simulink model "POWER_SYSTEM_FULL"  (R2025a)
settings: Solver=ode23t  StartTime=0  StopTime=5  FixedStep=1e-06  MinStep=1e-06  AbsTol=1e-6
model workspace (MAT data in the model file):
  CONTROL_INI.VSMP.PARAM.H = [15.5890205501 15.5890205501 15.5890205501 15.5890205501]
  CONTROL_INI.VSMP.PARAM.Dp = [20 20 20 20]
  CONTROL_INI.VSMP.PARAM.Dd = [0.156477821214 0.156477821214 0.156477821214 0.156477821214]
  CONTROL_INI.VSMP.PARAM.der2error = [1 1 1 1]
  CONTROL_INI.VSMP.TARGET.P_ref = [0.728496137496 0.728496137496 0.734176903563 0.734176903563]
  CONTROL_INI.VSMP.INPUT.P = [0.728496137496 0.728496137496 0.734176903563 0.734176903563]
  CONTROL_INI.VSMP.OUTPUT.w_pu = [1 1 1 1]
  CONTROL_INI.VSMP.OUTPUT.dth = [1 1 1 1]
  CONTROL_INI.VSMP.OUTPUT.th = [-0.655727257168 -0.655727257168 -0.596773515436 -0.596773515436]
  CONTROL_INI.VSMP.OUTPUT.MV = [20 20 20 20]
  CONTROL_INI.VSMP.STATE = [1  1  1  1; -0.655727257168  -0.655727257168  -0.596773515436  -0.596773515436]
  CONTROL_INI.VSMQ.PARAM.K_Fs_ref = [0.00177246709622 0.00177246709622 0.00177246709622 0.00177246709622]
  CONTROL_INI.VSMQ.PARAM.K_droopQV = [0.295235933108 0.295235933108 0.295235933108 0.295235933108]
  CONTROL_INI.VSMQ.TARGET.Vs_ref = [1 1 1 1]
  CONTROL_INI.VSMQ.TARGET.Q_ref = [0.279528149911 0.279528149911 0.34680626227 0.34680626227]
  CONTROL_INI.VSMQ.INPUT.Vs = [1.03097478396 1.03097478396 1.06643947684 1.06643947684]
  CONTROL_INI.VSMQ.INPUT.Q = [0.270383280666 0.270383280666 0.32719094133 0.32719094133]
  CONTROL_INI.VSMQ.OUTPUT.Fs_ref = [1.070537678 1.070537678 1.11055988863 1.11055988863]
  CONTROL_INI.VSMQ.OUTPUT.MV = [0 0 0 0]
  CONTROL_INI.VSMQ.STATE = [1.070537678 1.070537678 1.11055988863 1.11055988863]
  CONTROL_INI.RSCd.PARAM.Kp = [26.2007936931 26.2007936931 26.2007936931 26.2007936931]
  CONTROL_INI.RSCd.PARAM.Ki = [11667.9331248 11667.9331248 11667.9331248 11667.9331248]
  CONTROL_INI.RSCd.PARAM.b = [1 1 1 1]
  CONTROL_INI.RSCd.TARGET.iRSCd_ref = [1.07624735715 1.07624735715 1.16545801889 1.16545801889]
  CONTROL_INI.RSCd.INPUT.iRSCd = [1.07624735715 1.07624735715 1.16545801889 1.16545801889]
  CONTROL_INI.RSCd.OUTPUT.vRSCd = [0.0171862723129 0.0171862723129 0.0176580541869 0.0176580541869]
  CONTROL_INI.RSCd.OUTPUT.MV = [-0.00184970943607 -0.00184970943607 -0.00100750664806 -0.00100750664806]
  CONTROL_INI.RSCd.STATE = [-0.00184970943607 -0.00184970943607 -0.00100750664806 -0.00100750664806]
  CONTROL_INI.RSCq.PARAM.Kp = [26.9584626879 26.9584626879 26.9584626879 26.9584626879]
  CONTROL_INI.RSCq.PARAM.Ki = [11726.8571581 11726.8571581 11726.8571581 11726.8571581]
  CONTROL_INI.RSCq.PARAM.b = [1 1 1 1]
  CONTROL_INI.RSCq.TARGET.iRSCq_ref = [1.05756781089 1.05756781089 1.02646278241 1.02646278241]
  CONTROL_INI.RSCq.INPUT.iRSCq = [1.05756781089 1.05756781089 1.02646278241 1.02646278241]
  CONTROL_INI.RSCq.OUTPUT.vRSCq = [-0.142921611261 -0.142921611261 -0.1508739187 -0.1508739187]
  CONTROL_INI.RSCq.OUTPUT.MV = [-0.123549401898 -0.123549401898 -0.129680819521 -0.129680819521]
  CONTROL_INI.RSCq.STATE = [-0.123549401898 -0.123549401898 -0.129680819521 -0.129680819521]
  CONTROL_INI.VDC.PARAM.Kp = [0.0696845800453 0.0696845800453 0.0696845800453 0.0696845800453]
  CONTROL_INI.VDC.PARAM.Ki = [3.07602140958 3.07602140958 3.07602140958 3.07602140958]
  CONTROL_INI.VDC.PARAM.b = [1 1 1 1]
  CONTROL_INI.VDC.TARGET.Vdc2_ref = [1 1 1 1]
  CONTROL_INI.VDC.INPUT.Vdc2 = [1 1 1 1]
  CONTROL_INI.VDC.OUTPUT.Pg_ref = [-0.0767620514712 -0.0767620514712 -0.0776825582306 -0.0776825582306]
  CONTROL_INI.VDC.OUTPUT.MV = [-0.0767620514712 -0.0767620514712 -0.0776825582306 -0.0776825582306]
  CONTROL_INI.VDC.STATE = [-0.0767620514712 -0.0767620514712 -0.0776825582306 -0.0776825582306]
  CONTROL_INI.GSCd.PARAM.Kp = [0.322083043505 0.322083043505 0.322083043505 0.322083043505]
  CONTROL_INI.GSCd.PARAM.Ki = [127.577686075 127.577686075 127.577686075 127.577686075]
  CONTROL_INI.GSCd.PARAM.b = [1 1 1 1]
  CONTROL_INI.GSCd.TARGET.Qg_ref = [0 0 0 0]
  CONTROL_INI.GSCd.TARGET.iGSCd_ref = [0 0 0 0]
  CONTROL_INI.GSCd.INPUT.iGSCd = [-3.10168557505e-15 -3.10168557505e-15 -6.80011602583e-16 -6.80011602583e-16]
  CONTROL_INI.GSCd.OUTPUT.vGSCd = [0.0708413035779 0.0708413035779 0.0682389112282 0.0682389112282]
  CONTROL_INI.GSCd.OUTPUT.MV = [2.34814861689e-15 2.34814861689e-15 -1.1167396054e-15 -1.1167396054e-15]
  CONTROL_INI.GSCd.STATE = [2.34814861689e-15 2.34814861689e-15 -1.1167396054e-15 -1.1167396054e-15]
  CONTROL_INI.GSCq.PARAM.Kp = [0.336796601445 0.336796601445 0.336796601445 0.336796601445]
  CONTROL_INI.GSCq.PARAM.Ki = [112.607832611 112.607832611 112.607832611 112.607832611]
  CONTROL_INI.GSCq.PARAM.b = [1 1 1 1]
  CONTROL_INI.GSCq.TARGET.iGSCq_ref = [-0.128961227093 -0.128961227093 -0.126167626611 -0.126167626611]
  CONTROL_INI.GSCq.INPUT.iGSCq = [-0.128961227093 -0.128961227093 -0.126167626611 -0.126167626611]
  CONTROL_INI.GSCq.OUTPUT.vGSCq = [1.02862401667 1.02862401667 1.06435180834 1.06435180834]
  CONTROL_INI.GSCq.OUTPUT.MV = [-0.000289354764585 -0.000289354764585 -0.000283086666596 -0.000283086666596]
  CONTROL_INI.GSCq.STATE = [-0.000289354764585 -0.000289354764585 -0.000283086666596 -0.000283086666596]
  CONTROL_INI.VIMP.PARAM.Lv_pu = [0.06507 0.06507 0.06507 0.06507]
  CONTROL_INI.VIMP.PARAM.Rv_pu = [0 0 0 0]
  MODEL_INI.PARAM.SIM_SAMPLING_TIME = 1e-06
  MODEL_INI.PARAM.SIM_FINAL_TIME = 5
  MODEL_INI.BASE.Ub = 690
  MODEL_INI.BASE.Ib = 1760
  MODEL_INI.BASE.Sb = 2103402.50071
  MODEL_INI.BASE.Zb = 0.392045454545
  MODEL_INI.BASE.f0 = 50
  MODEL_INI.BASE.fbase = 50
  MODEL_INI.BASE.wbase = 314.159265359
  MODEL_INI.BASE.Lb = 0.00124791944015
  MODEL_INI.BASE.Cb = 0.00811920869106
  MODEL_INI.DFIG.PARAM.nDFIG = 4
  MODEL_INI.DFIG.PARAM.p = [2 2 2 2]
  MODEL_INI.DFIG.PARAM.WMECm = [157.079632679 157.079632679 157.079632679 157.079632679]
  MODEL_INI.DFIG.PARAM.WMECe = [314.159265359 314.159265359 314.159265359 314.159265359]
  MODEL_INI.DFIG.PARAM.Lsig_s_H = [8.7e-05 8.7e-05 8.7e-05 8.7e-05]
  MODEL_INI.DFIG.PARAM.Lsig_r_H = [8.7e-05 8.7e-05 8.7e-05 8.7e-05]
  MODEL_INI.DFIG.PARAM.Lm_H = [0.0025 0.0025 0.0025 0.0025]
  MODEL_INI.DFIG.PARAM.Ls_H = [0.002587 0.002587 0.002587 0.002587]
  MODEL_INI.DFIG.PARAM.Lr_H = [0.002587 0.002587 0.002587 0.002587]
  MODEL_INI.DFIG.PARAM.sigma = [0.0661284179513 0.0661284179513 0.0661284179513 0.0661284179513]
  MODEL_INI.DFIG.PARAM.Rs_Ohm = [0.0026 0.0026 0.0026 0.0026]
  MODEL_INI.DFIG.PARAM.Rr_Ohm = [0.0029 0.0029 0.0029 0.0029]
  MODEL_INI.DFIG.PARAM.Rc_Ohm = [1000000 1000000 1000000 1000000]
  MODEL_INI.DFIG.PARAM.Ur_open_rotor_V = [2070 2070 2070 2070]
  MODEL_INI.DFIG.PARAM.Cdc = [0.00225 0.00225 0.00225 0.00225]
  MODEL_INI.DFIG.PARAM.SCR_transformer = [10 10 5 5]
  MODEL_INI.DFIG.PARAM.XR_transformer = [10 10 10 10]
  MODEL_INI.DFIG.PARAM.Lt_H = [7.20486624699e-05 7.20486624699e-05 0.00014409732494 0.00014409732494]
  MODEL_INI.DFIG.PARAM.Rt_Ohm = [0.00226347548716 0.00226347548716 0.00452695097433 0.00452695097433]
  MODEL_INI.DFIG.PARAM.Lfgsc_H = [2.8e-05 2.8e-05 2.8e-05 2.8e-05]
  MODEL_INI.DFIG.PARAM.Rfgsc_Ohm = [0.000879645943005 0.000879645943005 0.000879645943005 0.000879645943005]
  MODEL_INI.DFIG.PARAM.Lsig_s_pu = [0.0697160387127 0.0697160387127 0.0697160387127 0.0697160387127]
  MODEL_INI.DFIG.PARAM.Lsig_r_pu = [0.0697160387127 0.0697160387127 0.0697160387127 0.0697160387127]
  MODEL_INI.DFIG.PARAM.Lm_pu = [2.00333444577 2.00333444577 2.00333444577 2.00333444577]
  MODEL_INI.DFIG.PARAM.Ls_pu = [2.07305048448 2.07305048448 2.07305048448 2.07305048448]
  MODEL_INI.DFIG.PARAM.Lr_pu = [2.07305048448 2.07305048448 2.07305048448 2.07305048448]
  MODEL_INI.DFIG.PARAM.sigma_pu = [0.0661284179513 0.0661284179513 0.0661284179513 0.0661284179513]
  MODEL_INI.DFIG.PARAM.Rs_pu = [0.00663188405797 0.00663188405797 0.00663188405797 0.00663188405797]
  MODEL_INI.DFIG.PARAM.Rr_pu = [0.00739710144928 0.00739710144928 0.00739710144928 0.00739710144928]
  MODEL_INI.DFIG.PARAM.Rc_pu = [2550724.63768 2550724.63768 2550724.63768 2550724.63768]
  MODEL_INI.DFIG.PARAM.Rfe_pu = [2550724.63768 2550724.63768 2550724.63768 2550724.63768]
  MODEL_INI.DFIG.PARAM.Ur_open_rotor_pu = [3 3 3 3]
  MODEL_INI.DFIG.PARAM.Cdc_pu = 0.483918802711
  MODEL_INI.DFIG.PARAM.Lt_pu = [0.057735026919 0.057735026919 0.115470053838 0.115470053838]
  MODEL_INI.DFIG.PARAM.Rt_pu = [0.0057735026919 0.0057735026919 0.0115470053838 0.0115470053838]
  MODEL_INI.DFIG.PARAM.Lfgsc_pu = [0.0224373457926 0.0224373457926 0.0224373457926 0.0224373457926]
  MODEL_INI.DFIG.PARAM.Rfgsc_pu = [0.00224373457926 0.00224373457926 0.00224373457926 0.00224373457926]
  MODEL_INI.DFIG.PARAM.J = [2.53 2.53 2.53 2.53]
  MODEL_INI.DFIG.PARAM.Jt_kgm2 = [800 800 800 800]
  MODEL_INI.DFIG.PARAM.Dt_Nms_rad = [0.1 0.1 0.1 0.1]
  MODEL_INI.DFIG.PARAM.Ktg_Nm_rad = [12500 12500 12500 12500]
  MODEL_INI.DFIG.PARAM.Dtg_Nms_rad = [130 130 130 130]
  MODEL_INI.DFIG.PARAM.Jg_kgm2 = [90 90 90 90]
  MODEL_INI.DFIG.PARAM.Dg_Nms_rad = [0.1 0.1 0.1 0.1]
  MODEL_INI.DFIG.PARAM.Ht_pu = [4.69220912201 4.69220912201 4.69220912201 4.69220912201]
  MODEL_INI.DFIG.PARAM.Dt_pu = [0.0011730522805 0.0011730522805 0.0011730522805 0.0011730522805]
  MODEL_INI.DFIG.PARAM.Hg_pu = [0.527873526226 0.527873526226 0.527873526226 0.527873526226]
  MODEL_INI.DFIG.PARAM.Dg_pu = [0.0011730522805 0.0011730522805 0.0011730522805 0.0011730522805]
  MODEL_INI.DFIG.PARAM.Dtg_pu = [1.52496796465 1.52496796465 1.52496796465 1.52496796465]
  MODEL_INI.DFIG.PARAM.Ktg_pu = [0.933485344735 0.933485344735 0.933485344735 0.933485344735]
  MODEL_INI.DFIG.PARAM.turbineData.ratedTurbinePower = 2000000
  MODEL_INI.DFIG.PARAM.turbineData.ratedTurbineSpeed = 2.80648943721
  MODEL_INI.DFIG.PARAM.turbineData.ratedWindSpeed = 12.5
  MODEL_INI.DFIG.PARAM.turbineData.turbineRadius = 35
  MODEL_INI.DFIG.PARAM.turbineData.airDensity = 1.225
  MODEL_INI.DFIG.PARAM.turbineData.Cp_coeff_matrix = [-0.533799944678  0.284966457097  -0.0246612463409  0.00070387634662  -6.19435778221e-06; 0.0502347840223  -0.0141180188397  0.000236959314197  9.72360914257e-05  -3.95863369447e-06; -0.0141053149856  0.00789606939988  -0.0013835145015  8.1445517726e-05  -1.33347929886e-06; 0.00189515235857  -0.00115030050123  0.000206019398382  -1.24987823414e-05  1.58554758305e-07; -7.04963027946e-05  4.2809340349e-05  -7.43463233727e-06  4.06348518101e-07  -2.85640254235e-09]
  MODEL_INI.DFIG.BASE.Udc_base = [1200 1200 1200 1200]
  MODEL_INI.DFIG.BASE.Idc_base = [1752.83541726 1752.83541726 1752.83541726 1752.83541726]
  MODEL_INI.DFIG.BASE.Zdc_base = [0.68460506228 0.68460506228 0.68460506228 0.68460506228]
  MODEL_INI.DFIG.BASE.Cdc_base = [0.00464954035139 0.00464954035139 0.00464954035139 0.00464954035139]
  MODEL_INI.DFIG.BASE.wmbase = [157.079632679 157.079632679 157.079632679 157.079632679]
  MODEL_INI.DFIG.BASE.Tebase = [13390.676212 13390.676212 13390.676212 13390.676212]
  MODEL_INI.DFIG.BASE.Jb = [85.2476924193 85.2476924193 85.2476924193 85.2476924193]
  MODEL_INI.DFIG.INPUT.vPCC_r = [0.714142842854 0.714142842854 0.714142842854 0.714142842854]
  MODEL_INI.DFIG.INPUT.vPCC_i = [0.7 0.7 0.7 0.7]
  MODEL_INI.DFIG.INPUT.vRSC_r = [-0.0735225072874 -0.0735225072874 -0.0701816981017 -0.0701816981017]
  MODEL_INI.DFIG.INPUT.vRSC_i = [-0.123759427292 -0.123759427292 -0.134719246855 -0.134719246855]
  MODEL_INI.DFIG.INPUT.vGSC_r = [0.683338070975 0.683338070975 0.654584845977 0.654584845977]
  MODEL_INI.DFIG.INPUT.vGSC_i = [0.772097752046 0.772097752046 0.842033253697 0.842033253697]
  MODEL_INI.DFIG.INPUT.windSpeed = [11.0080618911 11.0080618911 11.0368315613 11.0368315613]
  MODEL_INI.DFIG.INPUT.turbinePitch = [1 1 1 1]
  MODEL_INI.DFIG.OUTPUT.vs_r = [0.68545508048 0.68545508048 0.656767318105 0.656767318105]
  MODEL_INI.DFIG.OUTPUT.vs_i = [0.770104108417 0.770104108417 0.840208216834 0.840208216834]
  MODEL_INI.DFIG.OUTPUT.is_r = [-1.07438763375 -1.07438763375 -1.0821166602 -1.0821166602]
  MODEL_INI.DFIG.OUTPUT.is_i = [-0.50997333627 -0.50997333627 -0.507828664614 -0.507828664614]
  MODEL_INI.DFIG.OUTPUT.ir_r = [1.4978757059 1.4978757059 1.5408603146 1.5408603146]
  MODEL_INI.DFIG.OUTPUT.ir_i = [0.182006642923 0.182006642923 0.194081756892 0.194081756892]
  MODEL_INI.DFIG.OUTPUT.ig_r = [-0.0786322810944 -0.0786322810944 -0.0709032546372 -0.0709032546372]
  MODEL_INI.DFIG.OUTPUT.ig_i = [-0.102215275098 -0.102215275098 -0.104359946754 -0.104359946754]
  MODEL_INI.DFIG.OUTPUT.it_r = [1.15301991484 1.15301991484 1.15301991484 1.15301991484]
  MODEL_INI.DFIG.OUTPUT.it_i = [0.612188611368 0.612188611368 0.612188611368 0.612188611368]
  MODEL_INI.DFIG.OUTPUT.Vdc = [1 1 1 1]
  MODEL_INI.DFIG.OUTPUT.P_GSC = [-0.076587023214 -0.076587023214 -0.0775304863749 -0.0775304863749]
  MODEL_INI.DFIG.OUTPUT.P_RSC = [-0.0765870232066 -0.0765870232066 -0.0775304863727 -0.0775304863727]
  MODEL_INI.DFIG.OUTPUT.Pdc = [-7.36979921534e-12 -7.36979921534e-12 -2.18218498826e-12 -2.18218498826e-12]
  MODEL_INI.DFIG.OUTPUT.wr = [1.13130130564 1.13130130564 1.13264773079 1.13264773079]
  MODEL_INI.DFIG.OUTPUT.Pm = [0.746659273078 0.746659273078 0.752978959715 0.752978959715]
  MODEL_INI.DFIG.STATE = [0.706916556634  0.706916556634  0.710436806016  0.710436806016; -0.727925020657  -0.727925020657  -0.734633242246  -0.734633242246; 0.952814203022  0.952814203022  1.02643964198  1.02643964198; -0.644338191682  -0.644338191682  -0.615009376214  -0.615009376214; 1.13130130564  1.13130130564  1.13264773079  1.13264773079; 1  1  1  1; -0.0683339355027  -0.0683339355027  -0.134730152485  -0.134730152485; -0.0376381654294  -0.0376381654294  -0.0730310121258  -0.0730310121258; 1.13130130564  1.13130130564  1.13264773079  1.13264773079; 0.658673288027  0.658673288027  0.663466708323  0.663466708323]
  MODEL_INI.LINE.PARAM.nLINE = 1
  MODEL_INI.LINE.PARAM.R_pu = 1e-05
  MODEL_INI.LINE.PARAM.L_pu = 1e-05
  MODEL_INI.LINE.PARAM.Rn1_pu = 100
  MODEL_INI.LINE.PARAM.Cn1_pu = 0.001
  MODEL_INI.LINE.PARAM.Rn2_pu = 100
  MODEL_INI.LINE.PARAM.Cn2_pu = 0.001
  MODEL_INI.LINE.PARAM.load_node = 2
  MODEL_INI.LINE.INPUT.in1_r = 4.61207965936
  MODEL_INI.LINE.INPUT.in1_i = 2.44875444547
  MODEL_INI.LINE.INPUT.in2_r = 4.60563823093
  MODEL_INI.LINE.INPUT.in2_i = 2.44104030263
  MODEL_INI.LINE.INPUT.il1_r = 0
  MODEL_INI.LINE.INPUT.il1_i = 0
  MODEL_INI.LINE.INPUT.il2_r = 0
  MODEL_INI.LINE.INPUT.il2_i = 0
  MODEL_INI.LINE.OUTPUT.vn1_r = 0.714142842854
  MODEL_INI.LINE.OUTPUT.vn1_i = 0.7
  MODEL_INI.LINE.OUTPUT.Vpcc = 1
  MODEL_INI.LINE.OUTPUT.vn2_r = 1
  MODEL_INI.LINE.OUTPUT.vn2_i = 0
  MODEL_INI.LINE.OUTPUT.i_r = 4.60563823093
  MODEL_INI.LINE.OUTPUT.i_i = 2.44104030263
  MODEL_INI.LINE.STATE = [4.60563823093; 2.44104030263; 0.714142842854; 0.7; 1; 0]
  MODEL_INI.GRID.PARAM.nGRID = 1
  MODEL_INI.GRID.PARAM.SCR_grid = 1
  MODEL_INI.GRID.PARAM.XR_grid = 10
  MODEL_INI.GRID.PARAM.Lg_H = 0.000180121656175
  MODEL_INI.GRID.PARAM.Rg_Ohm = 0.00565868871791
  MODEL_INI.GRID.PARAM.Lg_pu = 0.144337567297
  MODEL_INI.GRID.PARAM.Rg_pu = 0.0144337567297
  MODEL_INI.GRID.PARAM.Deq_pu = 20
  MODEL_INI.GRID.PARAM.Tgov = 0.2
  MODEL_INI.GRID.PARAM.Ttb1 = 0.3
  MODEL_INI.GRID.PARAM.Ttb2 = 7
  MODEL_INI.GRID.PARAM.H = 5
  MODEL_INI.GRID.BASE.Ub = 690
  MODEL_INI.GRID.BASE.Sb = 8413610.00285
  MODEL_INI.GRID.INPUT.v_grid_r = 1
  MODEL_INI.GRID.INPUT.v_grid_i = 0
  MODEL_INI.GRID.INPUT.Pg_ref = -0.664766618104
  MODEL_INI.GRID.OUTPUT.f_pu = 1
  MODEL_INI.GRID.OUTPUT.Pmech = -0.664766618104
  MODEL_INI.GRID.OUTPUT.Pgrid = -0.664766618104
  MODEL_INI.GRID.OUTPUT.Qgrid = 0.352333818956
  MODEL_INI.GRID.STATE = [-0.664766618104; -0.664766618104; 0; 1]
  initialMemoryState = [1.15301991484; 1.15301991484; 1.15301991484; 1.15301991484; 0.612188611368; 0.612188611368; 0.612188611368; 0.612188611368; -1.07438763375; -1.07438763375; -1.0821166602; -1.0821166602; -0.50997333627; -0.50997333627; -0.507828664614; -0.507828664614; 1.4978757059; 1.4978757059; 1.5408603146; 1.5408603146; 0.182006642923; 0.182006642923; 0.194081756892; 0.194081756892; 0.68545508048; 0.68545508048; 0.656767318105; 0.656767318105; 0.770104108417; 0.770104108417; 0.840208216834; 0.840208216834; 1; 1; 1; 1; 1.13130130564; 1.13130130564; 1.13264773079; 1.13264773079]
undefined symbols (not defined in the file or in its folder): CONTROL, MODEL, monitorDFIG, pref_mask_vec, qref_mask_vec
(part 1 of 3)
settings SolverCC: SolverResetMethod=Robust
settings DataIOCC: LimitDataPoints=on  MaxDataPoints=1  SaveFinalState=on  SaveFormat=StructureWithTime  SaveOutput=off  SignalLogging=off  DSMLogging=off  SaveTime=off  ReturnWorkspaceOutputs=off
settings OptimizationCC: BlockReduction=off  OptimizeBlockIOStorage=off  BufferReuse=off
settings DebuggingCC: AlgebraicLoopMsg=none  ArtificialAlgebraicLoopMsg=none
settings ModelReferenceCC: EnableRefExpFcnMdlSchedulingChecks=on
settings RTWCC: GPUComputeCapability=3.5

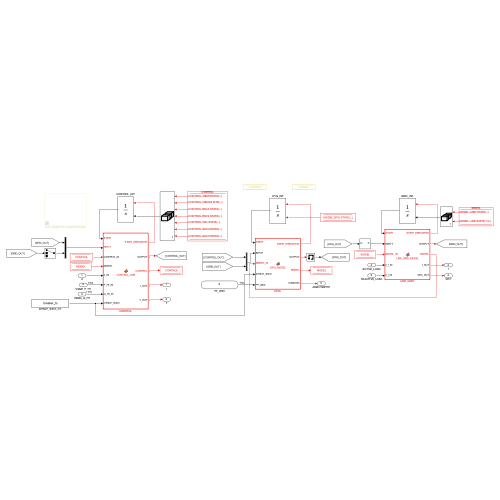
[thumbnail: Simulink's stored preview of the top-level diagram]
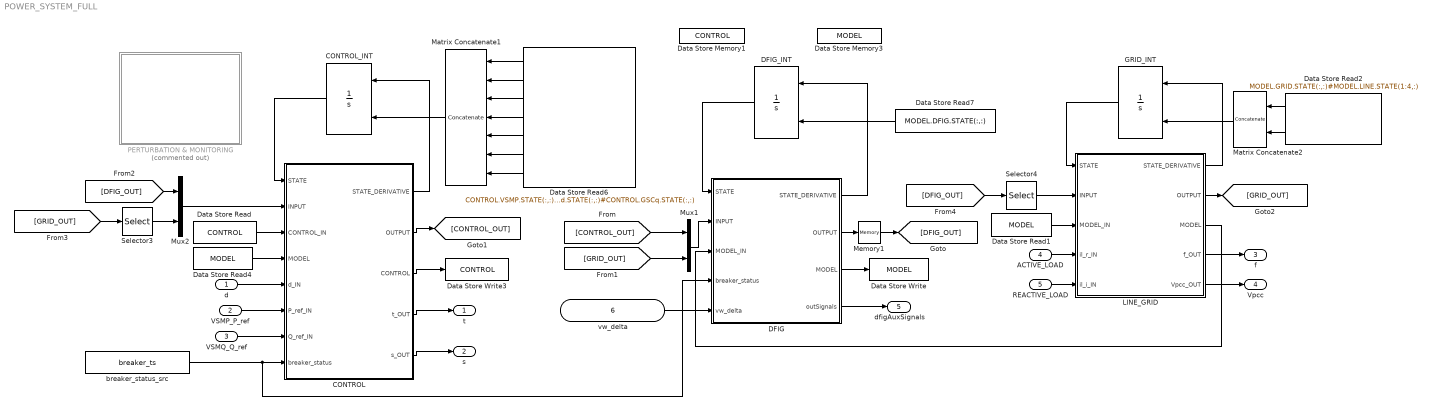
== system POWER_SYSTEM_FULL ==
  d : Inport
  VSMP_P_ref : Inport  Port=2  PortDimensions=[1 MODEL_INI.DFIG.PARAM.nDFIG]
  VSMQ_Q_ref : Inport  Port=3  PortDimensions=[1 MODEL_INI.DFIG.PARAM.nDFIG]
  ACTIVE_LOAD : Inport  Port=4  PortDimensions=1
  REACTIVE_LOAD : Inport  Port=5  PortDimensions=1
  vw_delta : Inport  Port=6  PortDimensions=[1 4]
  CONTROL : MATLAB Function  TreatAsAtomicUnit=on
  CONTROL_INT : Integrator  InitialConditionSource=external
  DFIG : MATLAB Function  TreatAsAtomicUnit=on
  DFIG_INT : Integrator  InitialConditionSource=external
  Data Store Memory1 : DataStoreMemory  Priority=2  DataStoreName=CONTROL  ReadBeforeWriteMsg=warning  WriteAfterWriteMsg=warning  WriteAfterReadMsg=warning  InitialValue=CONTROL_INI  ShowAdditionalParam=off  OutDataTypeStr=Bus: CONTROL_Bus
  Data Store Memory3 : DataStoreMemory  Priority=2  DataStoreName=MODEL  ReadBeforeWriteMsg=warning  WriteAfterWriteMsg=warning  WriteAfterReadMsg=warning  InitialValue=MODEL_INI  ShowAdditionalParam=off  OutDataTypeStr=Bus: MODEL_Bus
  Data Store Read : DataStoreRead  DataStoreName=CONTROL  IndexOptions=Index vector (dialog)  Indices=1  OutputSizes=1
  Data Store Read1 : DataStoreRead  DataStoreName=MODEL  IndexOptions=Index vector (dialog)  Indices=1  OutputSizes=1
  Data Store Read2 : DataStoreRead  DataStoreName=MODEL  DataStoreElements=MODEL.GRID.STATE(:,:)#MODEL.LINE.STATE(1:4,:)  IndexOptions=Index vector (dialog)  Indices=1  OutputSizes=1
  Data Store Read4 : DataStoreRead  DataStoreName=MODEL  IndexOptions=Index vector (dialog)  Indices=1  OutputSizes=1
  Data Store Read6 : DataStoreRead  DataStoreName=CONTROL  DataStoreElements=CONTROL.VSMP.STATE(:,:)#CONTROL.VSMQ.STATE(:,:)#CONTROL.RSCd.STATE(:,:)#CONTROL.RSCq.STATE(:,:)#CONTROL.VDC.STATE(:,:)#CONTROL.GSCd.STATE(:,:)#CONTROL.GSCq.STATE(:,:)  IndexOptions=Index vector (dialog)  Indices=1  OutputSizes=1
  Data Store Read7 : DataStoreRead  DataStoreName=MODEL  DataStoreElements=MODEL.DFIG.STATE(:,:)  IndexOptions=Index vector (dialog)  Indices=1  OutputSizes=1
  Data Store Write : DataStoreWrite  DataStoreName=MODEL  IndexOptions=Index vector (dialog)  Indices=1  OutputSizes=1
  Data Store Write3 : DataStoreWrite  DataStoreName=CONTROL  IndexOptions=Index vector (dialog)  Indices=1  OutputSizes=1
  GRID_INT : Integrator  InitialConditionSource=external
  LINE_GRID : MATLAB Function  TreatAsAtomicUnit=on
  Matrix Concatenate1 : Concatenate  NumInputs=7  Mode=Multidimensional array
  Matrix Concatenate2 : Concatenate  Mode=Multidimensional array
  Memory1 : Memory  InitialCondition=initialMemoryState  LinearizeMemory=on
  Mux1 : Mux  Inputs=2
  Mux2 : Mux  Inputs=2
  PERTURBATION & MONITORING : Subsystem  Priority=40  Commented=on
  Selector3 : Selector  InputPortWidth=3  IndexOptions=Index vector (dialog)  Indices=1  OutputSizes=1
  Selector4 : Selector  InputPortWidth=10*MODEL_INI.DFIG.PARAM.nDFIG  IndexOptions=Index vector (dialog)  Indices=1:8  OutputSizes=1
  breaker_status_src : FromWorkspace  VariableName=breaker_ts  Interpolate=off  OutputAfterFinalValue=Holding final value
  t : Outport
  s : Outport  Port=2
  f : Outport  Port=3
  Vpcc : Outport  Port=4
  dfigAuxSignals : Outport  Port=5
  wires:
  Data Store Read7/1 -> DFIG_INT/2
  DFIG_INT/1 -> DFIG/1(STATE)
  DFIG/1(STATE_DERIVATIVE) -> DFIG_INT/1
  DFIG/3(MODEL) -> Data Store Write/1
  GRID_INT/1 -> LINE_GRID/1(STATE)
  LINE_GRID/1(STATE_DERIVATIVE) -> GRID_INT/1
  CONTROL_INT/1 -> CONTROL/1(STATE)
  CONTROL/3(CONTROL) -> Data Store Write3/1
  Matrix Concatenate1/1 -> CONTROL_INT/2
  Data Store Read/1 -> CONTROL/3(CONTROL_IN)
  d/1 -> CONTROL/5(d_IN)
  CONTROL/4(t_OUT) -> t/1
  CONTROL/5(s_OUT) -> s/1
  Data Store Read6/1 -> Matrix Concatenate1/1
  Data Store Read6/2 -> Matrix Concatenate1/2
  Data Store Read6/3 -> Matrix Concatenate1/3
  Data Store Read6/4 -> Matrix Concatenate1/4
  Data Store Read6/5 -> Matrix Concatenate1/5
  Data Store Read6/6 -> Matrix Concatenate1/6
  Data Store Read6/7 -> Matrix Concatenate1/7
  VSMQ_Q_ref/1 -> CONTROL/7(Q_ref_IN)
  ACTIVE_LOAD/1 -> LINE_GRID/4(il_r_IN)
  REACTIVE_LOAD/1 -> LINE_GRID/5(il_i_IN)
  LINE_GRID/4(f_OUT) -> f/1
  LINE_GRID/5(Vpcc_OUT) -> Vpcc/1
  LINE_GRID/3(MODEL) -> DFIG/3(MODEL_IN)
  DFIG/2(OUTPUT) -> Memory1/1
  CONTROL/2(OUTPUT) -> [CONTROL_OUT]
  [CONTROL_OUT] -> Mux1/1
  [GRID_OUT] -> Mux1/2
  [DFIG_OUT] -> Mux2/1
  [GRID_OUT] -> Selector3/1
  Selector3/1 -> Mux2/2
  [DFIG_OUT] -> Selector4/1
  Data Store Read4/1 -> CONTROL/4(MODEL)
  Selector4/1 -> LINE_GRID/2(INPUT)
  Mux1/1 -> DFIG/2(INPUT)
  Mux2/1 -> CONTROL/2(INPUT)
  CONTROL/1(STATE_DERIVATIVE) -> CONTROL_INT/1
  LINE_GRID/2(OUTPUT) -> [GRID_OUT]
  Memory1/1 -> [DFIG_OUT]
  VSMP_P_ref/1 -> CONTROL/6(P_ref_IN)
  Data Store Read1/1 -> LINE_GRID/3(MODEL_IN)
  Data Store Read2/1 -> Matrix Concatenate2/1
  Data Store Read2/2 -> Matrix Concatenate2/2
  Matrix Concatenate2/1 -> GRID_INT/2
  DFIG/4(outSignals) -> dfigAuxSignals/1
  breaker_status_src/1 -> DFIG/4(breaker_status), CONTROL/8(breaker_status)
  vw_delta/1 -> DFIG/5(vw_delta)

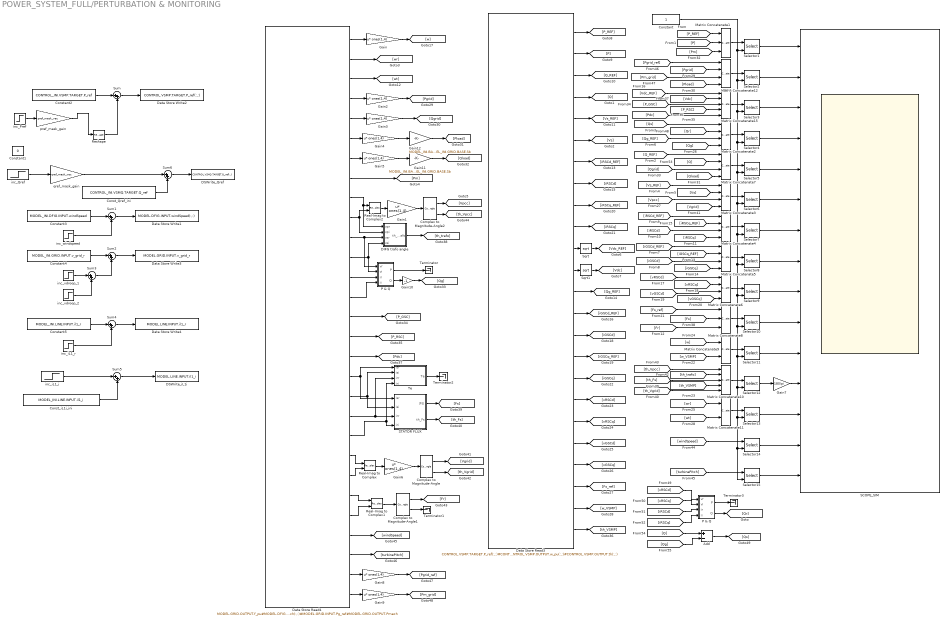
== system POWER_SYSTEM_FULL/PERTURBATION & MONITORING ==
  Add : Sum  Inputs=+-
  Complex to Magnitude-Angle : ComplexToMagnitudeAngle
  Complex to Magnitude-Angle1 : ComplexToMagnitudeAngle
  Complex to Magnitude-Angle2 : ComplexToMagnitudeAngle
  Const_Qref_ini : Constant  Value=CONTROL_INI.VSMQ.TARGET.Q_ref  SampleTime=-1
  Const_iL1i_ini : Constant  Value=MODEL_INI.LINE.INPUT.il1_i  SampleTime=-1
  Constant : Constant
  Constant1 : Constant  Value=0  VectorParams1D=off  SampleTime=-1
  Constant2 : Constant  Value=CONTROL_INI.VSMP.TARGET.P_ref  SampleTime=-1
  Constant3 : Constant  Value=MODEL_INI.DFIG.INPUT.windSpeed  SampleTime=-1
  Constant4 : Constant  Value=MODEL_INI.GRID.INPUT.v_grid_r  SampleTime=-1
  Constant5 : Constant  Value=MODEL_INI.LINE.INPUT.il1_r  SampleTime=-1
  DIFG trafo angle : Subsystem
  DSWrite_Qref : DataStoreWrite  DataStoreName=CONTROL  DataStoreElements=CONTROL.VSMQ.TARGET.Q_ref(:,:)  IndexOptions=Index vector (dialog)  Indices=1  OutputSizes=1
  DSWrite_iL1i : DataStoreWrite  DataStoreName=MODEL  DataStoreElements=MODEL.LINE.INPUT.il1_i  IndexOptions=Index vector (dialog)  Indices=1  OutputSizes=1
  Data Store Read3 : DataStoreRead  DataStoreName=CONTROL  DataStoreElements=CONTROL.VSMP.TARGET.P_ref(:,:)#CONTROL.VSMP.INPUT.P(:,:)#CONTROL.VSMQ.TARGET.Q_ref(:,:)#CONTROL.VSMQ.INPUT.Q(:,:)#CONTROL.VSMQ.TARGET.Vs_ref(:,:)#CONTROL.VSMQ.INPUT.Vs(:,:)#CONTROL.RSCd.TARGET.iRSCd_ref(:,:)#CONTROL.RSCd.INPUT.iRSCd(:,:)#CONTROL.RSCq.TARGET.iRSCq_ref(:,:)#CONTROL.RSCq.INPUT.iRSCq(:,:)#CONTROL.VDC.TARGET.Vdc2_ref(:,:)#CONTROL.VDC.INPUT.Vdc2(:,:)#CONTROL.GSCd.TARGET.Qg_ref(:,:)#CONTROL.GSCd.TARGET.iGSCd_ref(:,:)#CONTROL.GSCd.INPUT.iGSCd(:,:)#CONTROL.GSCq.TARGET.iGSCq_ref(:,:)#CONTROL.GSCq.INPUT.iGSCq(:,:)#CONTROL.RSCd.OUTPUT.vRSCd(:,:)#CONTROL.RSCq.OUTPUT.vRSCq(:,:)#CONTROL.GSCd.OUTPUT.vGSCd(:,:)#CONTROL.GSCq.OUTPUT.vGSCq(:,:)#CONTROL.VSMQ.OUTPUT.Fs_ref(:,:)#CONTROL.VSMP.OUTPUT.w_pu(:,:)#CONTROL.VSMP.OUTPUT.th(:,:)  IndexOptions=Index vector (dialog)  Indices=1  OutputSizes=1
  Data Store Read4 : DataStoreRead  DataStoreName=MODEL  DataStoreElements=MODEL.GRID.OUTPUT.f_pu#MODEL.DFIG.OUTPUT.wr(:,:)#MODEL.DFIG.STATE(9,:)#MODEL.GRID.OUTPUT.Pgrid#MODEL.GRID.OUTPUT.Qgrid#MODEL.LINE.INPUT.il1_r#MODEL.LINE.INPUT.il1_i#MODEL.DFIG.OUTPUT.Pm(:,:)#MODEL.LINE.OUTPUT.vn1_r#MODEL.LINE.OUTPUT.vn1_i#MODEL.DFIG.OUTPUT.vs_r(:,:)#MODEL.DFIG.OUTPUT.vs_i(:,:)#MODEL.DFIG.OUTPUT.ig_r(:,:)#MODEL.DFIG.OUTPUT.ig_i(:,:)#MODEL.DFIG.OUTPUT.P_GSC(:,:)#MODEL.DFIG.OUTPUT.P_RSC(:,:)#MODEL.DFIG.OUTPUT.Pdc(:,:)#MODEL.DFIG.OUTPUT.is_r(:,:)#MODEL.DFIG.OUTPUT.is_i(:,:)#MODEL.DFIG.OUTPUT.ir_r(:,:)#MODEL.DFIG.OUTPUT.ir_i(:,:)#MODEL.GRID.INPUT.v_grid_r#MODEL.GRID.INPUT.v_grid_i#MODEL.DFIG.STATE(3,:)#MODEL.DFIG.STATE(4,:)#MODEL.DFIG.INPUT.windSpeed(:,:)#MODEL.DFIG.INPUT.turbinePitch(:,:)#MODEL.GRID.INPUT.Pg_ref#MODEL.GRID.OUTPUT.Pmech  IndexOptions=Index vector (dialog)  Indices=1  OutputSizes=1
  Data Store Write1 : DataStoreWrite  DataStoreName=MODEL  DataStoreElements=MODEL.DFIG.INPUT.windSpeed(:,:)  IndexOptions=Index vector (dialog)  Indices=1  OutputSizes=1
  Data Store Write2 : DataStoreWrite  DataStoreName=CONTROL  DataStoreElements=CONTROL.VSMP.TARGET.P_ref(:,:)  IndexOptions=Index vector (dialog)  Indices=1  OutputSizes=1
  Data Store Write3 : DataStoreWrite  DataStoreName=MODEL  DataStoreElements=MODEL.GRID.INPUT.v_grid_r  IndexOptions=Index vector (dialog)  Indices=1  OutputSizes=1
  Data Store Write4 : DataStoreWrite  DataStoreName=MODEL  DataStoreElements=MODEL.LINE.INPUT.il1_r  IndexOptions=Index vector (dialog)  Indices=1  OutputSizes=1
  Gain{,1..6,8..9} (9 alike) : Gain  Gain=ones(1,4)  Multiplication=Matrix(u*K)
  Gain10 : Gain  Gain=-1
  Gain11 : Gain  Gain=MODEL_INI.BASE.Sb/MODEL_INI.GRID.BASE.Sb
  Gain12 : Gain  Gain=MODEL_INI.BASE.Sb/MODEL_INI.GRID.BASE.Sb
  Gain7 : Gain  Gain=180/pi
  Matrix Concatenate1 : Concatenate  NumInputs=3  Mode=Multidimensional array
  Matrix Concatenate10 : Concatenate  NumInputs=5  Mode=Multidimensional array
  Matrix Concatenate11 : Concatenate  Mode=Multidimensional array
  Matrix Concatenate{2..7,12} (7 alike) : Concatenate  NumInputs=4  Mode=Multidimensional array
  Matrix Concatenate15 : Concatenate  NumInputs=5  Mode=Multidimensional array
  Matrix Concatenate8 : Concatenate  NumInputs=3  Mode=Multidimensional array
  Matrix Concatenate9 : Concatenate  Mode=Multidimensional array
  P & Q : Subsystem
  "P & Q " : Subsystem
  Real-Imag to Complex : RealImagToComplex
  Real-Imag to Complex1 : RealImagToComplex
  Real-Imag to Complex2 : RealImagToComplex
  Reshape : Reshape  OutputDimensionality=Row vector (2-D)
  SCOPE_SIM : Scope  NumInputPorts=15
      settings: Title=DFIG ACTIVE POWER (pu)  ActiveDisplayYMinimum=0.70146460984873871  ActiveDisplayYMaximum=0.96691028131648715  DataLoggingVariableName=SCOPE_SIM
  STATOR FLUX : Subsystem
  Selector{1..15} (15 alike) : Selector  NumberOfDimensions=2  InputPortWidth=10  IndexOptions=Select all,Index vector (port)  Indices=monitorDFIG,1  OutputSizes=1,1
  Sqrt : Sqrt
  Sqrt1 : Sqrt
  Sum{,1..6} (7 alike) : Sum  Inputs=|++
  Te : Subsystem
  Terminator{,1..3} (4 alike) : Terminator
  inc_Pref : Step  After=0.2  SampleTime=0
  inc_Qref : Step  Time=999  After=0
  inc_iL1_i : Step  Time=999  After=0
  inc_iL1_r : Step  After=0.0  SampleTime=0
  inc_vdroop_1 : Step  After=0.0  SampleTime=0
  inc_vdroop_2 : Step  Time=1.5  After=0.0  SampleTime=0
  inc_windspeed : Step  After=0.0  SampleTime=0
  pref_mask_gain : Gain  Gain=pref_mask_vec
  qref_mask_gain : Gain  Gain=qref_mask_vec
  wires:
  Data Store Read3/2 -> [P]
  Data Store Read3/5 -> [Vs_REF]
  [P_REF] -> Matrix Concatenate1/1
  Data Store Read3/8 -> [iRSCd]
  Data Store Read3/4 -> [Q]
  Data Store Read3/7 -> [iRSCd_REF]
  Data Store Read3/6 -> [Vs]
  [P] -> Matrix Concatenate1/2
  Data Store Read3/9 -> [iRSCq_REF]
  Data Store Read3/10 -> [iRSCq]
  Data Store Read3/1 -> [P_REF]
  Data Store Read3/3 -> [Q_REF]
  Data Store Read3/11 -> Sqrt/1
  Data Store Read3/12 -> Sqrt1/1
  Data Store Read3/13 -> [Qg_REF]
  Data Store Read3/14 -> [iGSCd_REF]
  Data Store Read3/15 -> [iGSCd]
  Data Store Read3/16 -> [iGSCq_REF]
  Data Store Read3/17 -> [iGSCq]
  [Vs_REF] -> Matrix Concatenate3/1
  [Vs] -> Matrix Concatenate3/2
  [iRSCd_REF] -> Matrix Concatenate4/1
  Data Store Read3/18 -> [vRSCd]
  Data Store Read3/19 -> [vRSCq]
  Data Store Read3/20 -> [vGSCd]
  Data Store Read3/21 -> [vGSCq]
  Data Store Read3/22 -> [Fs_ref]
  Data Store Read3/23 -> [w_VSMP]
  Data Store Read3/24 -> [th_VSMP]
  Selector1/1 -> SCOPE_SIM/1
  Selector2/1 -> SCOPE_SIM/2
  Selector3/1 -> SCOPE_SIM/3
  Selector4/1 -> SCOPE_SIM/4
  Selector5/1 -> SCOPE_SIM/5
  Selector6/1 -> SCOPE_SIM/6
  Selector7/1 -> SCOPE_SIM/7
  Selector8/1 -> SCOPE_SIM/8
  Selector9/1 -> SCOPE_SIM/9
  Selector10/1 -> SCOPE_SIM/10
  Selector13/1 -> SCOPE_SIM/13
  Matrix Concatenate1/1 -> Selector1/1
  Data Store Read4/1 -> Gain/1
  Gain/1 -> [w]
  Data Store Read4/2 -> [wr]
  Gain2/1 -> [Pgrid]
  Gain3/1 -> [Qgrid]
  Gain4/1 -> Gain12/1
  [Vpcc] -> Matrix Concatenate3/3
  P & Q/1(P) -> Terminator/1
  P & Q/2(Q) -> Gain10/1
  STATOR FLUX/1(|Fs|) -> [Fs]
  STATOR FLUX/2(th_Fs) -> [th_Fs]
  Real-Imag to Complex/1 -> Gain6/1
  Complex to Magnitude-Angle/1 -> [Vgrid]
  Complex to Magnitude-Angle/2 -> [th_Vgrid]
  Complex to Magnitude-Angle1/2 -> Terminator1/1
  Complex to Magnitude-Angle1/1 -> [Fr]
  Real-Imag to Complex1/1 -> Complex to Magnitude-Angle1/1
  Data Store Read4/3 -> [wt]
  Data Store Read4/4 -> Gain2/1
  Data Store Read4/5 -> Gain3/1
  Data Store Read4/6 -> Gain4/1
  Data Store Read4/7 -> Gain5/1
  Data Store Read4/8 -> [Pm]
  [Vgrid] -> Matrix Concatenate3/4
  [iRSCq] -> Matrix Concatenate4/4
  Sqrt/1 -> [Vdc_REF]
  Sqrt1/1 -> [Vdc]
  Gain6/1 -> Complex to Magnitude-Angle/1
  Real-Imag to Complex2/1 -> Gain1/1
  Gain1/1 -> Complex to Magnitude-Angle2/1
  Complex to Magnitude-Angle2/1 -> [Vpcc]
  Complex to Magnitude-Angle2/2 -> [th_Vpcc]
  Data Store Read4/9 -> DIFG trafo angle/1(vpr), Real-Imag to Complex2/1
  Data Store Read4/10 -> DIFG trafo angle/2(vpi), Real-Imag to Complex2/2
  Data Store Read4/11 -> DIFG trafo angle/3(vsr), P & Q/1(vr)
  Data Store Read4/12 -> DIFG trafo angle/4(vsi), P & Q/2(vi)
  Data Store Read4/13 -> P & Q/3(ir)
  Data Store Read4/14 -> P & Q/4(ii)
  DIFG trafo angle/1(th_trafo) -> [th_trafo]
  Data Store Read4/15 -> [P_GSC]
  Data Store Read4/16 -> [P_RSC]
  Data Store Read4/17 -> [Pdc]
  Data Store Read4/24 -> Real-Imag to Complex1/1
  Data Store Read4/25 -> Real-Imag to Complex1/2
  Data Store Read4/22 -> Real-Imag to Complex/1
  Data Store Read4/23 -> Real-Imag to Complex/2
  Data Store Read4/18 -> STATOR FLUX/1(isr), Te/1(isr)
  Data Store Read4/19 -> STATOR FLUX/2(isi), Te/2(isi)
  Data Store Read4/20 -> Te/3(irr), STATOR FLUX/3(irr)
  Data Store Read4/21 -> Te/4(iri), STATOR FLUX/4(iri)
  [iGSCd_REF] -> Matrix Concatenate5/1
  [iGSCq] -> Matrix Concatenate5/4
  [vRSCd] -> Matrix Concatenate6/1
  [vRSCq] -> Matrix Concatenate6/2
  [vGSCd] -> Matrix Concatenate6/3
  [vGSCq] -> Matrix Concatenate6/4
  [Fs_ref] -> Matrix Concatenate8/1
  [Fs] -> Matrix Concatenate8/2
  [Fr] -> Matrix Concatenate8/3
  [w] -> Matrix Concatenate9/1
  [w_VSMP] -> Matrix Concatenate9/2
  [th_Vpcc] -> Matrix Concatenate10/1
  [th_trafo] -> Matrix Concatenate10/2
  [th_Fs] -> Matrix Concatenate10/3
  [th_VSMP] -> Matrix Concatenate10/4
  [th_Vgrid] -> Matrix Concatenate10/5
  [wr] -> Matrix Concatenate11/1
  [wt] -> Matrix Concatenate11/2
  Data Store Read4/26 -> [windSpeed]
  Selector11/1 -> SCOPE_SIM/11
  Selector12/1 -> Gain7/1
  Constant/1 -> Selector10/2, Selector15/2, Selector14/2, Selector13/2, Selector12/2, Selector11/2, Selector9/2, Selector8/2, Selector7/2, Selector6/2, Selector5/2, Selector4/2, Selector3/2, Selector2/2, Selector1/2
  Selector14/1 -> SCOPE_SIM/14
  Data Store Read4/27 -> [turbinePitch]
  [Pm] -> Matrix Concatenate1/3
  Data Store Read4/28 -> Gain8/1
  Data Store Read4/29 -> Gain9/1
  [Pgrid_ref] -> Matrix Concatenate12/1
  [Pgrid] -> Matrix Concatenate12/2
  [Pload] -> Matrix Concatenate12/4
  [Pm_grid] -> Matrix Concatenate12/3
  Matrix Concatenate15/1 -> Selector3/1
  Matrix Concatenate2/1 -> Selector4/1
  Matrix Concatenate7/1 -> Selector5/1
  Matrix Concatenate3/1 -> Selector6/1
  Matrix Concatenate4/1 -> Selector7/1
  Matrix Concatenate5/1 -> Selector8/1
  Matrix Concatenate6/1 -> Selector9/1
  Matrix Concatenate8/1 -> Selector10/1
  Matrix Concatenate9/1 -> Selector11/1
  Matrix Concatenate10/1 -> Selector12/1
  Matrix Concatenate11/1 -> Selector13/1
  [windSpeed] -> Selector14/1
  Selector15/1 -> SCOPE_SIM/15
  [turbinePitch] -> Selector15/1
  Gain8/1 -> [Pgrid_ref]
  Gain9/1 -> [Pm_grid]
  Matrix Concatenate12/1 -> Selector2/1
  [Vdc_REF] -> Matrix Concatenate15/1
  [Vdc] -> Matrix Concatenate15/2
  [P_GSC] -> Matrix Concatenate15/3
  [P_RSC] -> Matrix Concatenate15/4
  [Pdc] -> Matrix Concatenate15/5
  Constant2/1 -> Sum/1
  Reshape/1 -> Sum/2
  Sum/1 -> Data Store Write2/1
  Gain7/1 -> SCOPE_SIM/12
  Te/1(Te) -> Terminator2/1
  "P & Q "/1(P) -> Terminator3/1
  "P & Q "/2(Q) -> [Qr]
  Gain10/1 -> [Qg]
  [Q] -> Add/1
  [Qg] -> Add/2
  Add/1 -> [Qs]
  Gain5/1 -> Gain11/1
  Gain11/1 -> [Qload]
  Gain12/1 -> [Pload]
  [vRSCd] -> "P & Q "/1(vr)
  [vRSCq] -> "P & Q "/2(vi)
  [iRSCd] -> "P & Q "/3(ir)
  [iRSCq] -> "P & Q "/4(ii)
  [iRSCq_REF] -> Matrix Concatenate4/2
  [iRSCd] -> Matrix Concatenate4/3
  [iGSCq_REF] -> Matrix Concatenate5/2
  [iGSCd] -> Matrix Concatenate5/3
  [Q_REF] -> Matrix Concatenate7/1
  [Qload] -> Matrix Concatenate7/4
  [Qgrid] -> Matrix Concatenate7/3
  [Q] -> Matrix Concatenate7/2
  [Qg_REF] -> Matrix Concatenate2/3
  [Qg] -> Matrix Concatenate2/4
  [Qs] -> Matrix Concatenate2/1
  [Qr] -> Matrix Concatenate2/2
  Constant3/1 -> Sum1/1
  Sum1/1 -> Data Store Write1/1
  inc_windspeed/1 -> Sum1/2
  Sum2/1 -> Data Store Write3/1
  Constant4/1 -> Sum2/1
  inc_vdroop_1/1 -> Sum3/1
  Sum3/1 -> Sum2/2
  inc_vdroop_2/1 -> Sum3/2
  inc_iL1_r/1 -> Sum4/2
  Sum4/1 -> Data Store Write4/1
  Constant5/1 -> Sum4/1
  inc_Qref/1 -> qref_mask_gain/1
  qref_mask_gain/1 -> Sum6/1
  Const_Qref_ini/1 -> Sum6/2
  Sum6/1 -> DSWrite_Qref/1
  inc_iL1_i/1 -> Sum5/1
  Const_iL1i_ini/1 -> Sum5/2
  Sum5/1 -> DSWrite_iL1i/1
  inc_Pref/1 -> pref_mask_gain/1
  pref_mask_gain/1 -> Reshape/1

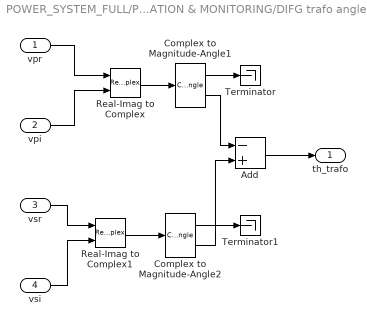
== system POWER_SYSTEM_FULL/PERTURBATION & MONITORING/DIFG trafo angle ==
  vpr : Inport
  vpi : Inport  Port=2
  vsr : Inport  Port=3
  vsi : Inport  Port=4
  Add : Sum  Inputs=-+
  Complex to Magnitude-Angle1 : ComplexToMagnitudeAngle
  Complex to Magnitude-Angle2 : ComplexToMagnitudeAngle
  Real-Imag to Complex : RealImagToComplex
  Real-Imag to Complex1 : RealImagToComplex
  Terminator : Terminator
  Terminator1 : Terminator
  th_trafo : Outport
  wires:
  vpr/1 -> Real-Imag to Complex/1
  vsr/1 -> Real-Imag to Complex1/1
  vsi/1 -> Real-Imag to Complex1/2
  vpi/1 -> Real-Imag to Complex/2
  Complex to Magnitude-Angle1/1 -> Terminator/1
  Add/1 -> th_trafo/1
  Real-Imag to Complex/1 -> Complex to Magnitude-Angle1/1
  Real-Imag to Complex1/1 -> Complex to Magnitude-Angle2/1
  Complex to Magnitude-Angle2/2 -> Add/2
  Complex to Magnitude-Angle1/2 -> Add/1
  Complex to Magnitude-Angle2/1 -> Terminator1/1

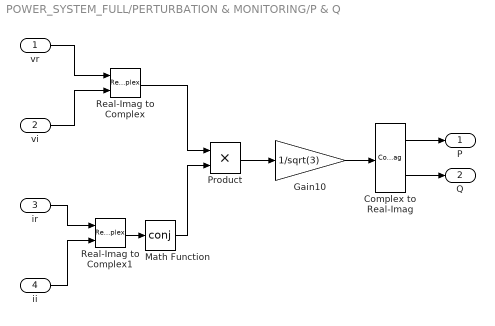
== system POWER_SYSTEM_FULL/PERTURBATION & MONITORING/P & Q ==
  vr : Inport
  vi : Inport  Port=2
  ir : Inport  Port=3
  ii : Inport  Port=4
  Complex to Real-Imag : ComplexToRealImag
  Gain10 : Gain  Gain=1/sqrt(3)
  Math Function : Math  Operator=conj
  Product : Product
  Real-Imag to Complex : RealImagToComplex
  Real-Imag to Complex1 : RealImagToComplex
  P : Outport
  Q : Outport  Port=2
  wires:
  Complex to Real-Imag/1 -> P/1
  vi/1 -> Real-Imag to Complex/2
  ii/1 -> Real-Imag to Complex1/2
  Complex to Real-Imag/2 -> Q/1
  ir/1 -> Real-Imag to Complex1/1
  vr/1 -> Real-Imag to Complex/1
  Real-Imag to Complex/1 -> Product/1
  Math Function/1 -> Product/2
  Product/1 -> Gain10/1
  Real-Imag to Complex1/1 -> Math Function/1
  Gain10/1 -> Complex to Real-Imag/1

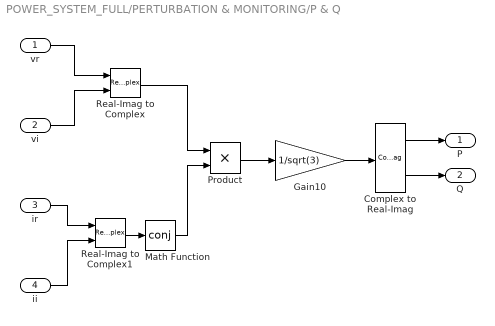
== system POWER_SYSTEM_FULL/PERTURBATION & MONITORING/P & Q  ==
  vr : Inport
  vi : Inport  Port=2
  ir : Inport  Port=3
  ii : Inport  Port=4
  Complex to Real-Imag : ComplexToRealImag
  Gain10 : Gain  Gain=1/sqrt(3)
  Math Function : Math  Operator=conj
  Product : Product
  Real-Imag to Complex : RealImagToComplex
  Real-Imag to Complex1 : RealImagToComplex
  P : Outport
  Q : Outport  Port=2
  wires:
  Complex to Real-Imag/1 -> P/1
  vi/1 -> Real-Imag to Complex/2
  ii/1 -> Real-Imag to Complex1/2
  Complex to Real-Imag/2 -> Q/1
  ir/1 -> Real-Imag to Complex1/1
  vr/1 -> Real-Imag to Complex/1
  Real-Imag to Complex/1 -> Product/1
  Math Function/1 -> Product/2
  Product/1 -> Gain10/1
  Real-Imag to Complex1/1 -> Math Function/1
  Gain10/1 -> Complex to Real-Imag/1

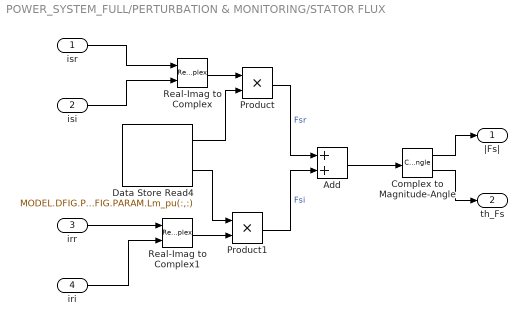
== system POWER_SYSTEM_FULL/PERTURBATION & MONITORING/STATOR FLUX ==
  isr : Inport
  isi : Inport  Port=2
  irr : Inport  Port=3
  iri : Inport  Port=4
  Add : Sum
  Complex to Magnitude-Angle : ComplexToMagnitudeAngle
  Data Store Read4 : DataStoreRead  DataStoreName=MODEL  DataStoreElements=MODEL.DFIG.PARAM.Ls_pu(:,:)#MODEL.DFIG.PARAM.Lm_pu(:,:)  IndexOptions=Index vector (dialog)  Indices=1  OutputSizes=1
  Product : Product
  Product1 : Product
  Real-Imag to Complex : RealImagToComplex
  Real-Imag to Complex1 : RealImagToComplex
  |Fs| : Outport
  th_Fs : Outport  Port=2
  wires:
  Real-Imag to Complex/1 -> Product/1
  irr/1 -> Real-Imag to Complex1/1
  isr/1 -> Real-Imag to Complex/1
  iri/1 -> Real-Imag to Complex1/2
  Complex to Magnitude-Angle/2 -> th_Fs/1
  Complex to Magnitude-Angle/1 -> |Fs|/1
  Product/1 -> Add/1  "Fsr"
  isi/1 -> Real-Imag to Complex/2
  Add/1 -> Complex to Magnitude-Angle/1
  Product1/1 -> Add/2  "Fsi"
  Real-Imag to Complex1/1 -> Product1/2
  Data Store Read4/1 -> Product/2
  Data Store Read4/2 -> Product1/1

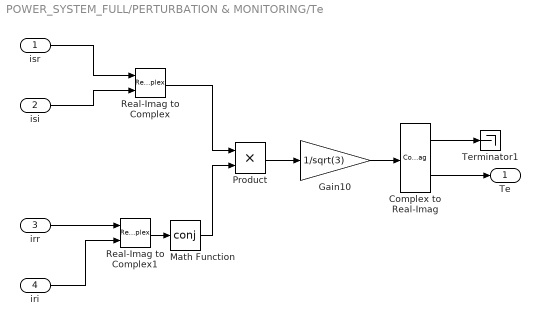
== system POWER_SYSTEM_FULL/PERTURBATION & MONITORING/Te ==
  isr : Inport
  isi : Inport  Port=2
  irr : Inport  Port=3
  iri : Inport  Port=4
  Complex to Real-Imag : ComplexToRealImag
  Gain10 : Gain  Gain=1/sqrt(3)
  Math Function : Math  Operator=conj
  Product : Product
  Real-Imag to Complex : RealImagToComplex
  Real-Imag to Complex1 : RealImagToComplex
  Terminator1 : Terminator
  Te : Outport
  wires:
  Complex to Real-Imag/2 -> Te/1
  Math Function/1 -> Product/2
  isr/1 -> Real-Imag to Complex/1
  isi/1 -> Real-Imag to Complex/2
  Real-Imag to Complex1/1 -> Math Function/1
  Real-Imag to Complex/1 -> Product/1
  Gain10/1 -> Complex to Real-Imag/1
  Product/1 -> Gain10/1
  irr/1 -> Real-Imag to Complex1/1
  iri/1 -> Real-Imag to Complex1/2
  Complex to Real-Imag/1 -> Terminator1/1
